simulink model "modelo_lti"  (R2022b)
settings: Solver=VariableStepAuto  StartTime=0.0  StopTime=10.0  RelTol=1e-3
values from neighbouring files (symbols this model uses):
  L_q = 5.8    [analisis_estabilidad.m]    (also in parametros.m = 0.0058; parametros_sim.m; polosyceros.m = L_q^3)
  R_s_ref = 1.02    [analisis_estabilidad.m]    (also in parametros.m; parametros_sim.m)
settings Model: Creator=martinarobyculasso  LastModifiedBy=martinarobyculasso

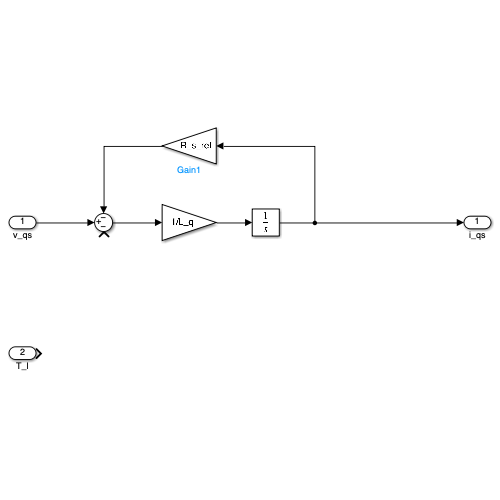
[thumbnail: Simulink's stored preview of the top-level diagram]
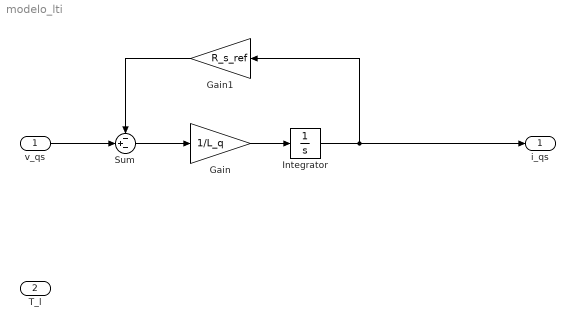
== system modelo_lti ==
  v_qs : Inport
  T_l : Inport  Port=2
  Gain : Gain  Gain=1/L_q
  Gain1 : Gain  Gain=R_s_ref
  Integrator : Integrator
  Sum : Sum  Inputs=-+-
  i_qs : Outport
  wires:
  v_qs/1 -> Sum/2
  Sum/1 -> Gain/1
  Gain/1 -> Integrator/1
  Gain1/1 -> Sum/1
  Integrator/1 -> i_qs/1, Gain1/1
